simulink model "oving2"  (R2023a)
settings: Solver=ode1  StartTime=0.0  StopTime=100  FixedStep=0.01  RelTol=1e-9  AbsTol=1e-9
undefined symbols (not defined in the file): a, b, c, d, f, g, h, i, j, k, l, m, n, o, p, rho, T, U, w, w1, w2, w3
libraries: simulink x19, mylib x1
settings Model: Creator=tormod  LastModifiedBy=redfox
settings DebuggingCC: UnconnectedInputMsg=warning  UnconnectedOutputMsg=warning  UnconnectedLineMsg=warning
settings ModelReferenceCC: EnableRefExpFcnMdlSchedulingChecks=on
settings RTWCC: DLArmComputeVersion=19.05

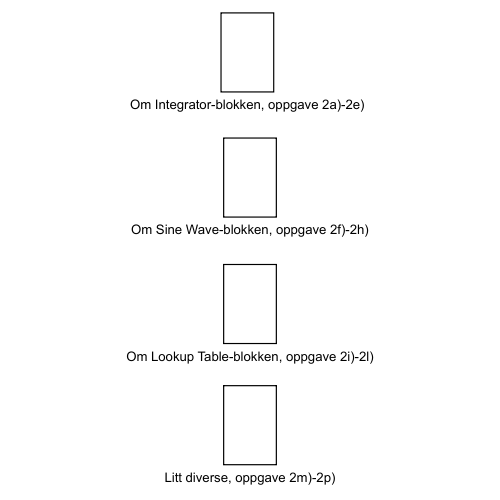
[thumbnail: Simulink's stored preview of the top-level diagram]
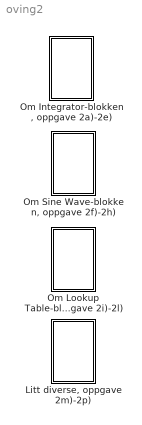
== system oving2 ==
  "Litt diverse, oppgave 2m)-2p)" : Subsystem
  "Om Integrator-blokken, oppgave 2a)-2e)" : Subsystem
  "Om Lookup Table-blokken, oppgave 2i)-2l)" : Subsystem
  "Om Sine Wave-blokken, oppgave 2f)-2h)" : Subsystem

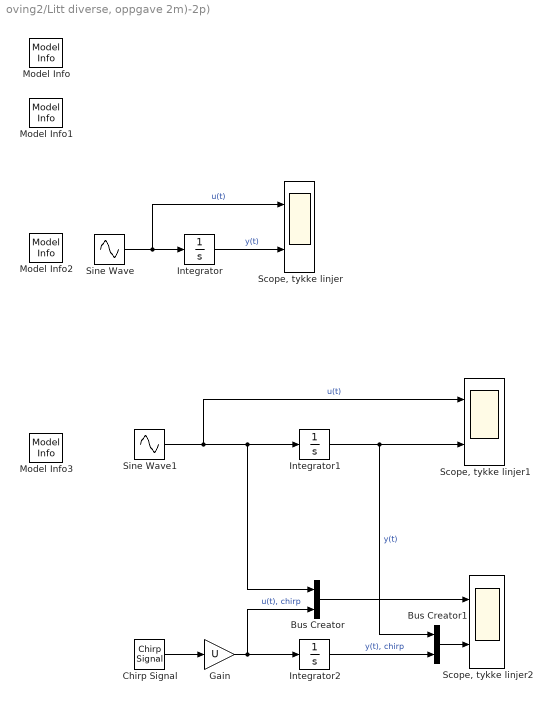
== system oving2/Litt diverse, oppgave 2m)-2p) ==
  Bus Creator : BusCreator  Inputs=2
  Bus Creator1 : BusCreator  Inputs=2
  Chirp Signal : simulink/Sources/Chirp Signal  f1=f1  T=100  f2=f3
      settings: AttributesFormatString=|
      | u(t) = sin(2 pi f(t) t)
      | f(t) = %<f1> + (%<f2>-%<f1>)/%<T>*t   [Hz]
  Gain : Gain  Gain=U
  Integrator : Integrator  InitialCondition=-pi/2
      settings: AttributesFormatString=IC = %<InitialCondition>
  Integrator1 : Integrator  InitialCondition=[-U/w1, -U/w2, -U/w3]
      settings: AttributesFormatString=IC = %<InitialCondition>
  Integrator2 : Integrator  InitialCondition=-U/w1
      settings: AttributesFormatString=IC = %<InitialCondition>
  Model Info : simulink/Model-Wide Utilities/Model Info  Frame=on  DisplayStringWithTags=m)  HorizontalTextAlignment=Center  LeftAlignmentValue=0.5
  Model Info1 : simulink/Model-Wide Utilities/Model Info  Frame=on  DisplayStringWithTags=n)  HorizontalTextAlignment=Center  LeftAlignmentValue=0.5
  Model Info2 : simulink/Model-Wide Utilities/Model Info  Frame=on  DisplayStringWithTags=o)  HorizontalTextAlignment=Center  LeftAlignmentValue=0.5
  Model Info3 : simulink/Model-Wide Utilities/Model Info  Frame=on  DisplayStringWithTags=p)  HorizontalTextAlignment=Center  LeftAlignmentValue=0.5
  "Scope, tykke linjer" : Scope  NumInputPorts=2
  "Scope, tykke linjer1" : Scope  NumInputPorts=2
  "Scope, tykke linjer2" : Scope  NumInputPorts=2
  Sine Wave : Sin  Amplitude=U  Frequency=w  SampleTime=0
      settings: AttributesFormatString=u(t) = %<Amplitude> sin(%<Frequency>t + %<Phase>) + %<Bias>
  Sine Wave1 : Sin  Amplitude=U  Frequency=[w1 w2 w3]  SampleTime=0
      settings: AttributesFormatString=u(t) = %<Amplitude> sin(%<Frequency>t + %<Phase>) + %<Bias>
  wires:
  Sine Wave/1 -> "Scope, tykke linjer"/1, Integrator/1  "u(t)"
  Integrator/1 -> "Scope, tykke linjer"/2  "y(t)"
  Integrator1/1 -> Bus Creator1/1, "Scope, tykke linjer1"/2  "y(t)"
  Sine Wave1/1 -> "Scope, tykke linjer1"/1, Bus Creator/1, Integrator1/1  "u(t)"
  Chirp Signal/1 -> Gain/1
  Gain/1 -> Bus Creator/2, Integrator2/1  "u(t), chirp"
  Bus Creator/1 -> "Scope, tykke linjer2"/1
  Integrator2/1 -> Bus Creator1/2  "y(t), chirp"
  Bus Creator1/1 -> "Scope, tykke linjer2"/2

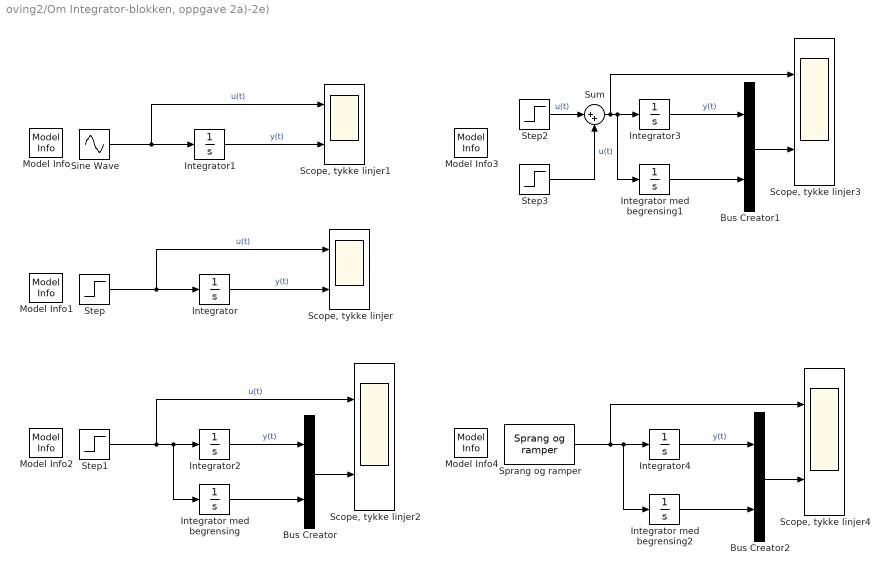
== system oving2/Om Integrator-blokken, oppgave 2a)-2e) ==
  Bus Creator : BusCreator  Inputs=2
  Bus Creator1 : BusCreator  Inputs=2
  Bus Creator2 : BusCreator  Inputs=2
  Integrator{,2..4} (4 alike) : Integrator  InitialCondition=-20
      settings: AttributesFormatString=IC = %<InitialCondition>
  Integrator med begrensing : Integrator  InitialCondition=-20  LimitOutput=on  UpperSaturationLimit=30
      settings: AttributesFormatString=|
      | IC = %<InitialCondition>
      | Max = %<UpperSaturationLimit>
      | Min = %<LowerSaturationLimit>
  Integrator med begrensing1 : Integrator  InitialCondition=-20  LimitOutput=on  UpperSaturationLimit=30
      settings: AttributesFormatString=|
      | IC = %<InitialCondition>
      | Max = %<UpperSaturationLimit>
      | Min = %<LowerSaturationLimit>
  Integrator med begrensing2 : Integrator  InitialCondition=-20  LimitOutput=on  UpperSaturationLimit=30
      settings: AttributesFormatString=|
      | IC = %<InitialCondition>
      | Max = %<UpperSaturationLimit>
      | Min = %<LowerSaturationLimit>
  Integrator1 : Integrator
      settings: AttributesFormatString=IC = %<InitialCondition>
  Model Info : simulink/Model-Wide Utilities/Model Info  Frame=on  DisplayStringWithTags=a)  HorizontalTextAlignment=Center  LeftAlignmentValue=0.5
  Model Info1 : simulink/Model-Wide Utilities/Model Info  Frame=on  DisplayStringWithTags=b)  HorizontalTextAlignment=Center  LeftAlignmentValue=0.5
  Model Info2 : simulink/Model-Wide Utilities/Model Info  Frame=on  DisplayStringWithTags=c)  HorizontalTextAlignment=Center  LeftAlignmentValue=0.5
  Model Info3 : simulink/Model-Wide Utilities/Model Info  Frame=on  DisplayStringWithTags=d)  HorizontalTextAlignment=Center  LeftAlignmentValue=0.5
  Model Info4 : simulink/Model-Wide Utilities/Model Info  Frame=on  DisplayStringWithTags=e)  HorizontalTextAlignment=Center  LeftAlignmentValue=0.5
  Scope, tykke linjer{,1..4} (5 alike) : Scope  NumInputPorts=2
  Sine Wave : Sin  Amplitude=2  Frequency=5  SampleTime=0
      settings: AttributesFormatString=u(t) = %<Amplitude> sin(%<Frequency>t + %<Phase>) + %<Bias>
  Sprang og ramper : mylib/ELE130/Sprang og ramper  tidspunkt=[0 5 10 15 20]  utgangsverdi=[0 4 0 -5 2]  valg=Linear
      settings: SourceProductName=Eget bibliotek
      settings: AttributesFormatString=|
      | t = %<tidspunkt>
      | u = %<utgangsverdi>
  Step : Step  Time=5  After=4  SampleTime=0
      settings: AttributesFormatString=|
      | u(t) = %<Before> for t < %<Time>s
      |       = %<After> for t > %<Time>s
  Step1 : Step  Time=5  After=4  SampleTime=0
      settings: AttributesFormatString=|
      | u(t) = %<Before> for t < %<Time>s
      |       = %<After> for t > %<Time>s
  Step2 : Step  Time=5  After=4  SampleTime=0
      settings: AttributesFormatString=|
      | u(t) = %<Before> for t < %<Time>s
      |       = %<After> for t > %<Time>s
  Step3 : Step  Time=13  After=-4  SampleTime=0
      settings: AttributesFormatString=|
      | u(t) = %<Before> for t < %<Time>s
      |       = %<After> for t > %<Time>s
  Sum : Sum  Inputs=|++
  wires:
  Step/1 -> "Scope, tykke linjer"/1, Integrator/1  "u(t)"
  Integrator/1 -> "Scope, tykke linjer"/2  "y(t)"
  Integrator1/1 -> "Scope, tykke linjer1"/2  "y(t)"
  Sine Wave/1 -> "Scope, tykke linjer1"/1, Integrator1/1  "u(t)"
  Integrator2/1 -> Bus Creator/1  "y(t)"
  Step1/1 -> "Scope, tykke linjer2"/1, Integrator med begrensing/1, Integrator2/1  "u(t)"
  Bus Creator/1 -> "Scope, tykke linjer2"/2
  Integrator med begrensing/1 -> Bus Creator/2
  Integrator3/1 -> Bus Creator1/1  "y(t)"
  Bus Creator1/1 -> "Scope, tykke linjer3"/2
  Integrator med begrensing1/1 -> Bus Creator1/2
  Step2/1 -> Sum/1  "u(t)"
  Step3/1 -> Sum/2  "u(t)"
  Sum/1 -> "Scope, tykke linjer3"/1, Integrator med begrensing1/1, Integrator3/1
  Integrator4/1 -> Bus Creator2/1  "y(t)"
  Bus Creator2/1 -> "Scope, tykke linjer4"/2
  Integrator med begrensing2/1 -> Bus Creator2/2
  Sprang og ramper/1 -> "Scope, tykke linjer4"/1, Integrator med begrensing2/1, Integrator4/1

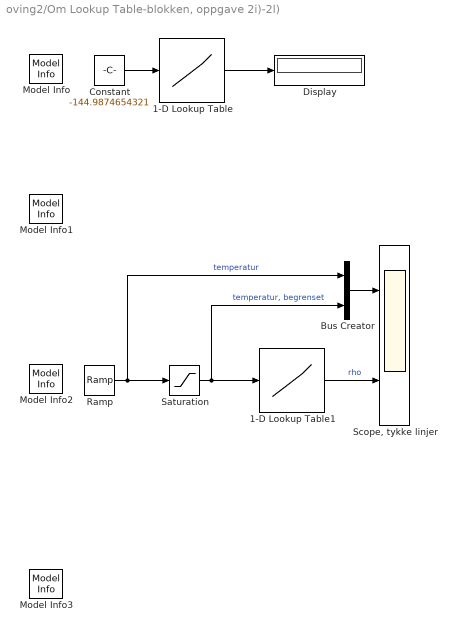
== system oving2/Om Lookup Table-blokken, oppgave 2i)-2l) ==
  1-D Lookup Table : Lookup_n-D  NumberOfTableDimensions=1  BreakpointsForDimension1=T  Table=rho  InternalRulePriority=Speed  RndMeth=Simplest
      settings: AttributesFormatString=|
      | INN = %<BreakpointsForDimension1>
      | UT = %<Table>
  1-D Lookup Table1 : Lookup_n-D  NumberOfTableDimensions=1  BreakpointsForDimension1=T  Table=rho  InternalRulePriority=Speed  RndMeth=Simplest
      settings: AttributesFormatString=|
      | INN = %<BreakpointsForDimension1>
      | UT = %<Table>
  Bus Creator : BusCreator  Inputs=2
  Constant : Constant  Value=-144.9874654321
  Display : Display
  Model Info : simulink/Model-Wide Utilities/Model Info  Frame=on  DisplayStringWithTags=i)  HorizontalTextAlignment=Center  LeftAlignmentValue=0.5
  Model Info1 : simulink/Model-Wide Utilities/Model Info  Frame=on  DisplayStringWithTags=j)  HorizontalTextAlignment=Center  LeftAlignmentValue=0.5
  Model Info2 : simulink/Model-Wide Utilities/Model Info  Frame=on  DisplayStringWithTags=k)  HorizontalTextAlignment=Center  LeftAlignmentValue=0.5
  Model Info3 : simulink/Model-Wide Utilities/Model Info  Frame=on  DisplayStringWithTags=l)  HorizontalTextAlignment=Center  LeftAlignmentValue=0.5
  Ramp : simulink/Sources/Ramp  slope=16  start=0  InitialOutput=-200
      settings: AttributesFormatString="u(t) = %<InitialOutput>  + %<slope> (t - %<start>)"
  Saturation : Saturate  UpperLimit=100  LowerLimit=-150
      settings: AttributesFormatString=|
      | Max = %<UpperLimit>
      | Min = %<LowerLimit>
  "Scope, tykke linjer" : Scope  NumInputPorts=2
  wires:
  Constant/1 -> 1-D Lookup Table/1
  1-D Lookup Table/1 -> Display/1
  1-D Lookup Table1/1 -> "Scope, tykke linjer"/2  "rho"
  Saturation/1 -> 1-D Lookup Table1/1, Bus Creator/2  "temperatur, begrenset"
  Ramp/1 -> Saturation/1, Bus Creator/1  "temperatur"
  Bus Creator/1 -> "Scope, tykke linjer"/1

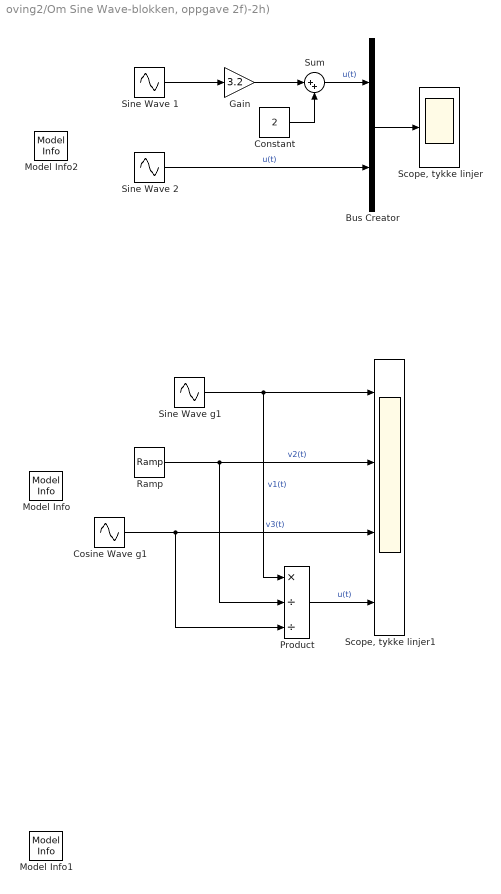
== system oving2/Om Sine Wave-blokken, oppgave 2f)-2h) ==
  Bus Creator : BusCreator  Inputs=2
  Constant : Constant  Value=2
  Cosine Wave g1 : Sin  Amplitude=1.7  Bias=3  Frequency=0.7  Phase=pi/2  SampleTime=0
      settings: AttributesFormatString=u(t) = %<Amplitude> sin(%<Frequency>t + %<Phase>) + %<Bias>
  Gain : Gain  Gain=3.2
  Model Info : simulink/Model-Wide Utilities/Model Info  Frame=on  DisplayStringWithTags=g)  HorizontalTextAlignment=Center  LeftAlignmentValue=0.5
  Model Info1 : simulink/Model-Wide Utilities/Model Info  Frame=on  DisplayStringWithTags=h)  HorizontalTextAlignment=Center  LeftAlignmentValue=0.5
  Model Info2 : simulink/Model-Wide Utilities/Model Info  Frame=on  DisplayStringWithTags=f)  HorizontalTextAlignment=Center  LeftAlignmentValue=0.5
  Product : Product  Inputs=*//
  Ramp : simulink/Sources/Ramp  slope=0.3  start=15  InitialOutput=1
      settings: AttributesFormatString="u(t) = %<InitialOutput>  + %<slope> (t - %<start>)"
  "Scope, tykke linjer" : Scope
  "Scope, tykke linjer1" : Scope  NumInputPorts=4
  Sine Wave 1 : Sin  Frequency=1.2  SampleTime=0
      settings: AttributesFormatString=u(t) = %<Amplitude> sin(%<Frequency>t + %<Phase>) + %<Bias>
  Sine Wave 2 : Sin  Amplitude=3.2  Bias=2  Frequency=1.2  SampleTime=0
      settings: AttributesFormatString=u(t) = %<Amplitude> sin(%<Frequency>t + %<Phase>) + %<Bias>
  Sine Wave g1 : Sin  Amplitude=3.2  Bias=2  Frequency=1.2  SampleTime=0
      settings: AttributesFormatString=u(t) = %<Amplitude> sin(%<Frequency>t + %<Phase>) + %<Bias>
  Sum : Sum  Inputs=|++
  wires:
  Sine Wave 1/1 -> Gain/1
  Gain/1 -> Sum/1
  Constant/1 -> Sum/2
  Sum/1 -> Bus Creator/1  "u(t)"
  Bus Creator/1 -> "Scope, tykke linjer"/1
  Sine Wave 2/1 -> Bus Creator/2  "u(t)"
  Cosine Wave g1/1 -> Product/3, "Scope, tykke linjer1"/3  "v3(t)"
  Ramp/1 -> Product/2, "Scope, tykke linjer1"/2  "v2(t)"
  Product/1 -> "Scope, tykke linjer1"/4  "u(t)"
  Sine Wave g1/1 -> Product/1, "Scope, tykke linjer1"/1  "v1(t)"
